simulink model "wheel1"  (R2014a)
settings: Solver=ode45  StartTime=0.0  StopTime=5.0  FixedStep=0.001  RelTol=1e-3
StartFcn:
  | wCoeff=[2.0703e6; -4.38e4; 0; 0]
values from neighbouring files (symbols this model uses):
  B1 = 0.01    [FinalProject.m]
  Bm = 0.005    [FinalProject.m]
  dc = 3.5    [FinalProject.m]
  Jm = 5e-4    (= 0.0005)    [FinalProject.m]
  Jw = 1e-3    (= 0.001)    [FinalProject.m]
  m1 = 0.9/32    (= 0.028125)    [FinalProject.m]
  m2 = 2.6/32    (= 0.08125)    [FinalProject.m]
  m3 = 0.9/32    (= 0.028125)    [FinalProject.m]
  mc = 4.4/32    (= 0.1375)    [FinalProject.m]
  N = 1    [FinalProject.m]
  tArray = [0 tArray]    [FinalProject.m]
libraries: simulink x1
settings Model: Creator=collinsjm  LastModifiedBy=collinsjm

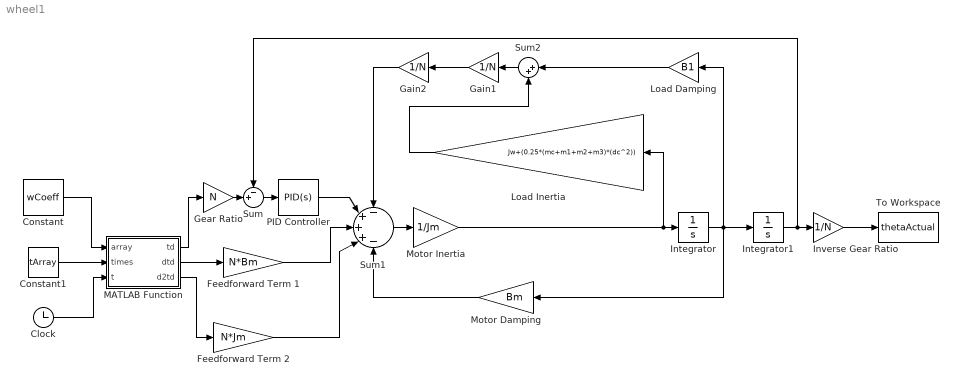
== system wheel1 ==
  Clock : Clock
  Constant : Constant  Value=wCoeff
  Constant1 : Constant  Value=tArray
  Feedforward Term 1 : Gain  Gain=N*Bm
  Feedforward Term 2 : Gain  Gain=N*Jm
  Gain1 : Gain  Gain=1/N
  Gain2 : Gain  Gain=1/N
  Gear Ratio : Gain  Gain=N
  Integrator : Integrator
  Integrator1 : Integrator
  Inverse Gear Ratio : Gain  Gain=1/N
  Load Damping : Gain  Gain=B1
  Load Inertia : Gain  Gain=Jw+(0.25*(mc+m1+m2+m3)*(dc^2))
  MATLAB Function : MATLAB Function  TreatAsAtomicUnit=on
  Motor Damping : Gain  Gain=Bm
  Motor Inertia : Gain  Gain=1/Jm
  PID Controller : simulink/Continuous/PID Controller  Controller=PID  TimeDomain=Continuous-time  SampleTime=1  IntegratorMethod=Forward Euler  FilterMethod=Forward Euler  Form=Parallel  P=125  I=25  D=10  N=100  InitialConditionSource=internal  InitialConditionForIntegrator=0  InitialConditionForFilter=0  ExternalReset=none  LimitOutput=off  UpperSaturationLimit=inf  LowerSaturationLimit=-inf  LinearizeAsGain=on  AntiWindupMode=none  Kb=1  TrackingMode=off  Kt=1  PParamMin=[]  PParamMax=[]  IParamMin=[]  IParamMax=[]  DParamMin=[]  DParamMax=[]  NParamMin=[]  NParamMax=[]  KbParamMin=[]  KbParamMax=[]  KtParamMin=[]  KtParamMax=[]  POutMin=[]  POutMax=[]  IOutMin=[]  IOutMax=[]  DOutMin=[]  DOutMax=[]  NOutMin=[]  NOutMax=[]  KbOutMin=[]  KbOutMax=[]  KtOutMin=[]  KtOutMax=[]  IntegratorOutMin=[]  IntegratorOutMax=[]  FilterOutMin=[]  FilterOutMax=[]  SumOutMin=[]  SumOutMax=[]  SumI1OutMin=[]  SumI1OutMax=[]  SumI2OutMin=[]  SumI2OutMax=[]  SumI3OutMin=[]  SumI3OutMax=[]  SumDOutMin=[]  SumDOutMax=[]  SaturationOutMin=[]  SaturationOutMax=[]  IntegratorContinuousStateAttributes=''  IntegratorStateMustResolveToSignalObject=off  IntegratorRTWStateStorageClass=Auto  FilterContinuousStateAttributes=''  FilterStateMustResolveToSignalObject=off  FilterRTWStateStorageClass=Auto
  Sum : Sum  Inputs=-+|
  Sum1 : Sum  Inputs=-+++-
  Sum2 : Sum  Inputs=|++
  To Workspace : ToWorkspace  VariableName=thetaActual  SaveFormat=Timeseries  SampleTime=-1
  wires:
  Clock/1 -> MATLAB Function/3(t)
  MATLAB Function/1(td) -> Gear Ratio/1
  Gear Ratio/1 -> Sum/2
  Sum/1 -> PID Controller/1
  Sum1/1 -> Motor Inertia/1
  Motor Inertia/1 -> Load Inertia/1, Integrator/1
  Integrator/1 -> Load Damping/1, Integrator1/1, Motor Damping/1
  PID Controller/1 -> Sum1/2
  Motor Damping/1 -> Sum1/5
  Load Damping/1 -> Sum2/1
  Load Inertia/1 -> Sum2/2
  Sum2/1 -> Gain1/1
  Gain1/1 -> Gain2/1
  Gain2/1 -> Sum1/1
  MATLAB Function/2(dtd) -> Feedforward Term 1/1
  Feedforward Term 1/1 -> Sum1/3
  MATLAB Function/3(d2td) -> Feedforward Term 2/1
  Feedforward Term 2/1 -> Sum1/4
  Constant/1 -> MATLAB Function/1(array)
  Integrator1/1 -> Inverse Gear Ratio/1, Sum/1
  Constant1/1 -> MATLAB Function/2(times)
  Inverse Gear Ratio/1 -> To Workspace/1

== matlab function wheel1/MATLAB Function ==
  data: array input; times input; td output; t input; dtd output; d2td output
function [td,dtd,d2td] = thetaD(array,times,t)
n=find(t <= times);
if length(n) == 0
    n = length(times);
else
    n = n(1);
end

a2 = array(n,:);

td=polyval(a2,t);

ad=polyder(a2);
dtd=polyval(ad,t);

ad2=polyder(ad);
d2td=polyval(ad2,t);
end
